simulink model "piv_dc_motor"  (R2022b)
settings: Solver=FixedStepAuto  StartTime=0.0  StopTime=50  FixedStep=T  RelTol=1e-3
values from neighbouring files (symbols this model uses):
  AW = 1 / T    (= 10)    [piv.m]    (also in uro_exp.m)
  I = 11.3341    [piv.m]    (also in uro_exp.m)
  P = 0.588235    [piv.m]    (also in uro_exp.m)
  u_max = 0.7    [piv.m]    (also in uro_exp.m)
  u_min = -0.7    [piv.m]    (also in uro_exp.m)
  V = 6.00043    [piv.m]    (also in uro_exp.m)
libraries: cstblocks x3
settings Model: Creator=ladislav  LastModifiedBy=ladislav

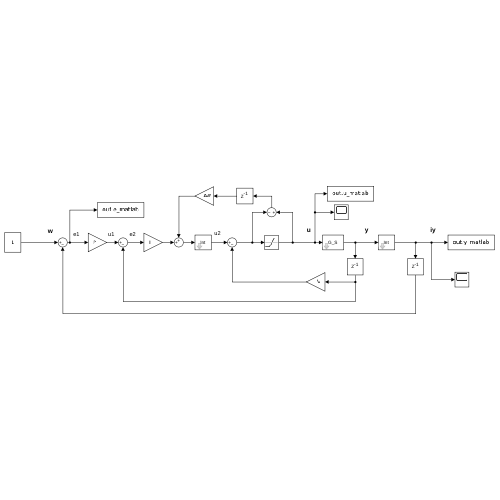
[thumbnail: Simulink's stored preview of the top-level diagram]
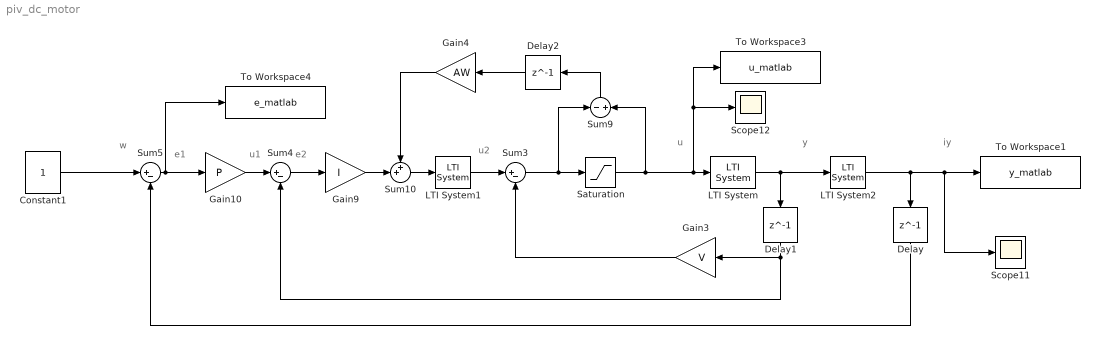
== system piv_dc_motor ==
  note: w
  note: iy
  note: u
  note: u2
  note: e1
  note: e2
  note: u1
  note: y
  Constant1 : Constant
  Delay : Delay  DelayLength=1
  Delay1 : Delay  DelayLength=1
  Delay2 : Delay  DelayLength=1
  Gain10 : Gain  Gain=P
  Gain3 : Gain  Gain=V
  Gain4 : Gain  Gain=AW
  Gain9 : Gain  Gain=I
  LTI System : cstblocks/LTI System  sys=G_S  IC=[]
  LTI System1 : cstblocks/LTI System  sys=Int  IC=[]
  LTI System2 : cstblocks/LTI System  sys=Int  IC=[]
  Saturation : Saturate  UpperLimit=u_max  LowerLimit=u_min  LinearizeAsGain=off
  Scope11 : Scope
  Scope12 : Scope
  Sum10 : Sum  Inputs=++|
  Sum3 : Sum  Inputs=|+-
  Sum4 : Sum  Inputs=|+-
  Sum5 : Sum  Inputs=|+-
  Sum9 : Sum  Inputs=-|+
  To Workspace1 : ToWorkspace  VariableName=y_matlab  SaveFormat=Timeseries  SampleTime=-1
  To Workspace3 : ToWorkspace  VariableName=u_matlab  SaveFormat=Timeseries  SampleTime=-1
  To Workspace4 : ToWorkspace  VariableName=e_matlab  SaveFormat=Timeseries  SampleTime=-1
  wires:
  Sum5/1 -> To Workspace4/1, Gain10/1
  Gain3/1 -> Sum3/2
  LTI System/1 -> LTI System2/1, Delay1/1
  LTI System1/1 -> Sum3/1
  Sum3/1 -> Sum9/1, Saturation/1
  Gain10/1 -> Sum4/1
  Constant1/1 -> Sum5/1
  LTI System2/1 -> Scope11/1, To Workspace1/1, Delay/1
  Sum4/1 -> Gain9/1
  Sum10/1 -> LTI System1/1
  Gain9/1 -> Sum10/2
  Sum9/1 -> Delay2/1
  Delay/1 -> Sum5/2
  Delay1/1 -> Sum4/2, Gain3/1
  Saturation/1 -> Sum9/2, LTI System/1, To Workspace3/1, Scope12/1
  Gain4/1 -> Sum10/1
  Delay2/1 -> Gain4/1
